simulink model "Autonomous_sort_of_working"  (R2019b)
settings: Solver=FixedStepAuto  StartTime=0.0  StopTime=inf  RelTol=1e-3
libraries: vexarmcortexlib x5, vexcommonlib x1
settings Model: ExtModeTrigDuration=25  Creator=nicoa  LastModifiedBy=nicoa
settings OptimizationCC: EnhancedBackFolding=on  PassReuseOutputArgsAs=Individual arguments  ZeroExternalMemoryAtStartup=off  ZeroInternalMemoryAtStartup=off  MaxStackSize=64  OptimizeBlockOrder=speed  DifferentSizesBufferReuse=on  OptimizationCustomize=off  EfficientTunableParamExpr=on
settings DebuggingCC: ParameterTunabilityLossMsg=error
settings HardwareCC: ProdBitPerPointer=32  ProdBitPerSizeT=32  ProdBitPerPtrDiffT=32  ProdLargestAtomicInteger=Long  ProdLargestAtomicFloat=Double  ProdWordSize=32  ProdHWDeviceType=ARM Compatible->ARM Cortex
settings SFSimCC: MATLABDynamicMemAlloc=off
settings RTWCC: SystemTargetFile=ert.tlc  HardwareBoard=ARM Cortex-based VEX Microcontroller  TLCOptions="-aInlineSetEventsForThisBaseRateFcn=TLC_FALSE -aSuppressMultiTaskScheduler=TLC_FALSE  -aRateBasedStepFcn=0"  TemplateMakefile=ert_default_tmf  GenerateReport=on  Toolchain=GNU Tools for VEX ARM Cortex  IncludeHyperlinkInReport=on  LaunchReport=on  GenerateTraceInfo=on  GenerateTraceReport=on  GenerateTraceReportSl=on  GenerateTraceReportSf=on  GenerateTraceReportEml=on
settings CodeAppCC: ForceParamTrailComments=on  IgnoreCustomStorageClasses=off  OperatorAnnotations=on  SimulinkDataObjDesc=on  SFDataObjDesc=on  InsertBlockDesc=on
settings ERTTargetCC: ExtMode=on  ExtModeTransport=1  ExtModeMexFile=ext_serial_win32_comm  ExtModeMexArgs=1 5 115200

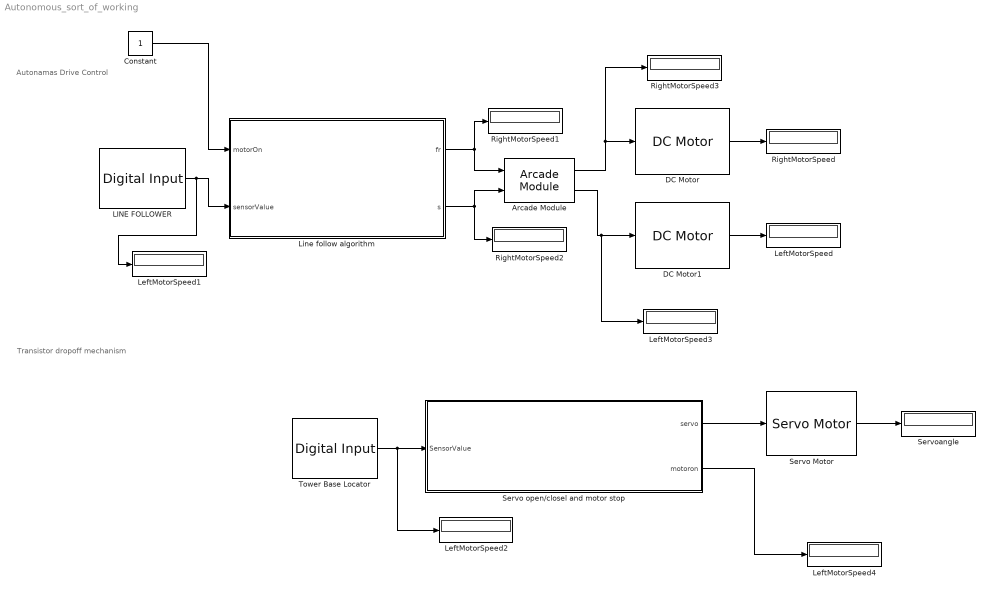
== system Autonomous_sort_of_working ==
  note: Transistor dropoff mechanism
  note: Autonamas Drive Control
  Arcade Module : vexcommonlib/Arcade Module  BlockPlatform=vexarmcortex
      settings: SourceProductName=Simulink Coder Support Package for ARM Cortex-based VEX Microcontroller  SourceProductBaseCode=EC_VEX_MICRO
  Constant : Constant
  DC Motor : vexarmcortexlib/Actuators/DC Motor  motor=2  scaleFactor=1/13.5  SimulationOut=on
      settings: SourceProductName=Simulink Coder Support Package for ARM Cortex-based VEX Microcontroller  SourceProductBaseCode=EC_VEX_MICRO
  DC Motor1 : vexarmcortexlib/Actuators/DC Motor  motor=9  scaleFactor=1/13.5  SimulationOut=on
      settings: SourceProductName=Simulink Coder Support Package for ARM Cortex-based VEX Microcontroller  SourceProductBaseCode=EC_VEX_MICRO
  LINE FOLLOWER : vexarmcortexlib/Sensors/Digital Input  inChan=1  SimulationIn=off  SampleTime=0.2
      settings: SourceProductName=Simulink Coder Support Package for ARM Cortex-based VEX Microcontroller  SourceProductBaseCode=EC_VEX_MICRO
  LeftMotorSpeed{,1..4} (5 alike) : Display
  Line follow algorithm : Stateflow chart  TreatAsAtomicUnit=on
  RightMotorSpeed{,1..3} (4 alike) : Display
  Servo Motor : vexarmcortexlib/Actuators/Servo Motor  motor=3  scaleFactor=60/127  SimulationOut=on
      settings: SourceProductName=Simulink Coder Support Package for ARM Cortex-based VEX Microcontroller  SourceProductBaseCode=EC_VEX_MICRO
  Servo open/closel and motor stop : Stateflow chart  TreatAsAtomicUnit=on
  Servoangle : Display
  Tower Base Locator : vexarmcortexlib/Sensors/Digital Input  inChan=11  SimulationIn=off  SampleTime=0.2
      settings: SourceProductName=Simulink Coder Support Package for ARM Cortex-based VEX Microcontroller  SourceProductBaseCode=EC_VEX_MICRO
  wires:
  Servo open/closel and motor stop/1(servo) -> Servo Motor/1
  Tower Base Locator/1 -> LeftMotorSpeed2/1, Servo open/closel and motor stop/1(SensorValue)
  LINE FOLLOWER/1 -> LeftMotorSpeed1/1, Line follow algorithm/2(sensorValue)
  DC Motor/1 -> RightMotorSpeed/1
  DC Motor1/1 -> LeftMotorSpeed/1
  Servo Motor/1 -> Servoangle/1
  Constant/1 -> Line follow algorithm/1(motorOn)
  Line follow algorithm/2(s) -> RightMotorSpeed2/1, Arcade Module/2
  Line follow algorithm/1(fr) -> RightMotorSpeed1/1, Arcade Module/1
  Arcade Module/1 -> RightMotorSpeed3/1, DC Motor/1
  Arcade Module/2 -> LeftMotorSpeed3/1, DC Motor1/1
  Servo open/closel and motor stop/2(motoron) -> LeftMotorSpeed4/1

== stateflow chart Autonomous_sort_of_working/Line follow algorithm ==
  state GO_RIGHT
    entry:
    fr = -20;
    s = 20;
  state GO_LEFT
    entry:
    fr = -20;
    s = -20;
  state STOPPED
    entry:
    fr = 0;
    s = 0;
  (default) -> GO_LEFT
  GO_LEFT -> GO_RIGHT [order 2] : [sensorValue == 0]
  GO_RIGHT -> GO_LEFT [order 2] : [sensorValue == 1]
  GO_LEFT -> STOPPED [order 1] : [motorOn == 0]
  GO_RIGHT -> STOPPED [order 1] : [motorOn == 0]
  data: fr output; s output; motorOn input; sensorValue input

== stateflow chart Autonomous_sort_of_working/Servo open//closel and motor stop ==
  state move
    entry:
    servo = 0;
    motoron = 1;
  state Stop
    entry:
    servo = 67;
    motoron = 0;
  state off
    entry:
    servo = 0;
    motoron = 0;
  (default) -> move
  move -> Stop : [SensorValue == 1]
  Stop -> off : [after(4,sec)]
  data: SensorValue input; servo output; motoron output
